simulink model "DDCU_wxt_v02_forA_OpenLoop"  (R2014a)
settings: Solver=FixedStepDiscrete  StartTime=0.0  StopTime=16  FixedStep=0.05  RelTol=1e-3
InitFcn:
  | Veh_Par_wxt
values from neighbouring files (symbols this model uses):
  ag_thr = 0.4*g    (= 3.924)    [Veh_Par_wxt.m]
  B = 2.25    [Veh_Par_wxt.m]
  bra_pre_em = 12    [Veh_Par_wxt.m]
  bra_pre_gz2 = 12/3    (= 4)    [Veh_Par_wxt.m]
  bra_pre_gz34 = 12/3    (= 4)    [Veh_Par_wxt.m]
  bra_pre_yd = 12/2    (= 6)    [Veh_Par_wxt.m]
  brakepre_dem_data = [0 1 2 3 4 5 6 7 8 9 10 11 12]    [Veh_Par_wxt.m]
  brakeTrq_dem_data = [0 218.198 436.396 654.594 872.792 1090.99 1309.188 1527.386 1745.584 1963.782 2181.98 2400.178 2618.376]    [Veh_Par_wxt.m]
  bratrq_max = 4*2618.376    (= 10473.504)    [Veh_Par_wxt.m]
  eff_tran = 0.75    [Veh_Par_wxt.m]
  G = Mass*g    (= 36297)    [Veh_Par_wxt.m]
  kd1 = 1    [Veh_Par_wxt.m]
  kd2 = 1    [Veh_Par_wxt.m]
  kd3 = 1    [Veh_Par_wxt.m]
  ki1 = 1    [Veh_Par_wxt.m]
  ki2 = 1    [Veh_Par_wxt.m]
  ki3 = 1    [Veh_Par_wxt.m]
  kp1 = 1    [Veh_Par_wxt.m]
  kp2 = 1    [Veh_Par_wxt.m]
  kp3 = 1    [Veh_Par_wxt.m]
  L = 3.12    [Veh_Par_wxt.m]
  premax = 12    [Veh_Par_wxt.m]
  Radius = 0.20    (= 0.2)    [Veh_Par_wxt.m]
  s_opt_yi_add = 0.05    [Veh_Par_wxt.m]
  s_opt_zhuan_add = 0.05    [Veh_Par_wxt.m]
  spd_map_mot = [0 100 200 300 360 400 500 600 700 800 900]*tras_ratio    [Veh_Par_wxt.m]
  spdmax = 900*tras_ratio    (= 5580)    [Veh_Par_wxt.m]
  speed_thr_park = 5/3.6/Radius*30/pi    (= 66.3145596216)    [Veh_Par_wxt.m]
  tras_ratio = 6.2    [Veh_Par_wxt.m]
  trq_map_mot = [1200 1200 1200 1200 1200 1080 864 720 617 540 480]/tras_ratio    [Veh_Par_wxt.m]
  trqmax = 80    [Veh_Par_wxt.m]
  v_thr1_b = 5    [Veh_Par_wxt.m]
  v_thr2_b = 20    [Veh_Par_wxt.m]
  v_thr_park = 5    [Veh_Par_wxt.m]
undefined symbols (not defined in the file or in its folder): DiscIntNeverNeededParam, sigbuilder_block
libraries: simulink x169, ec5744lib x9
(part 3 of 13)

== system DDCU_wxt_v02_forA_OpenLoop/OutputSignalProcess/VCU_ESC/VVMS_BrkPSetLe_MPa ==
  VVMS_BrkPSetLe_MPa : Inport
  Constant{2..8} (7 alike) : Constant  Value=0  OutDataTypeStr=uint8
  VVMS_BrkPSetLe_MPaRon : Rounding  Operator=round
  VVMS_BrkPSetLe_MPa_1sat : Saturate  UpperLimit=255  LowerLimit=0
  VVMS_BrkPSetLe_MPa_Convert : DataTypeConversion  OutDataTypeStr=uint8
  VVMS_BrkPSetLe_MPa_Convert1 : DataTypeConversion  OutDataTypeStr=uint32
  VVMS_BrkPSetLe_MPa_D : Product  Inputs=*/
  VVMS_BrkPSetLe_MPa_F : Constant  Value=0.1  OutDataTypeStr=single
  VVMS_BrkPSetLe_MPa_L : simulink/Logic and Bit Operations/Bitwise Operator  logicop=AND  UseBitMask=on  BitMask=255  BitMaskRealWorld=Stored Integer
  VVMS_BrkPSetLe_MPa_O : Constant  Value=0  OutDataTypeStr=single
  VVMS_BrkPSetLe_MPa_S : ArithShift
  VVMS_BrkPSetLe_MPa_sat : Saturate  UpperLimit=25.5  LowerLimit=0
  VVMS_BrkPSetLe_MPa_st : Sum  Inputs=+-
  output1 : Outport
  output2 : Outport  Port=2
  output3 : Outport  Port=3
  output4 : Outport  Port=4
  output5 : Outport  Port=5
  output6 : Outport  Port=6
  output7 : Outport  Port=7
  output8 : Outport  Port=8
  wires:
  VVMS_BrkPSetLe_MPa/1 -> VVMS_BrkPSetLe_MPa_sat/1
  VVMS_BrkPSetLe_MPa_sat/1 -> VVMS_BrkPSetLe_MPa_st/1
  VVMS_BrkPSetLe_MPa_O/1 -> VVMS_BrkPSetLe_MPa_st/2
  VVMS_BrkPSetLe_MPa_st/1 -> VVMS_BrkPSetLe_MPa_D/1
  VVMS_BrkPSetLe_MPa_F/1 -> VVMS_BrkPSetLe_MPa_D/2
  VVMS_BrkPSetLe_MPa_D/1 -> VVMS_BrkPSetLe_MPaRon/1
  VVMS_BrkPSetLe_MPaRon/1 -> VVMS_BrkPSetLe_MPa_S/1
  VVMS_BrkPSetLe_MPa_S/1 -> VVMS_BrkPSetLe_MPa_1sat/1
  VVMS_BrkPSetLe_MPa_1sat/1 -> VVMS_BrkPSetLe_MPa_Convert1/1
  VVMS_BrkPSetLe_MPa_Convert1/1 -> VVMS_BrkPSetLe_MPa_L/1
  VVMS_BrkPSetLe_MPa_L/1 -> VVMS_BrkPSetLe_MPa_Convert/1
  VVMS_BrkPSetLe_MPa_Convert/1 -> output1/1
  Constant2/1 -> output2/1
  Constant3/1 -> output3/1
  Constant4/1 -> output4/1
  Constant5/1 -> output5/1
  Constant6/1 -> output6/1
  Constant7/1 -> output7/1
  Constant8/1 -> output8/1

== system DDCU_wxt_v02_forA_OpenLoop/OutputSignalProcess/VCU_ESC/VVMS_BrkPSetRi_MPa ==
  VVMS_BrkPSetRi_MPa : Inport
  Constant{1,3..8} (7 alike) : Constant  Value=0  OutDataTypeStr=uint8
  VVMS_BrkPSetRi_MPaRon : Rounding  Operator=round
  VVMS_BrkPSetRi_MPa_1sat : Saturate  UpperLimit=255  LowerLimit=0
  VVMS_BrkPSetRi_MPa_Convert : DataTypeConversion  OutDataTypeStr=uint8
  VVMS_BrkPSetRi_MPa_Convert1 : DataTypeConversion  OutDataTypeStr=uint32
  VVMS_BrkPSetRi_MPa_D : Product  Inputs=*/
  VVMS_BrkPSetRi_MPa_F : Constant  Value=0.1  OutDataTypeStr=single
  VVMS_BrkPSetRi_MPa_L : simulink/Logic and Bit Operations/Bitwise Operator  logicop=AND  UseBitMask=on  BitMask=255  BitMaskRealWorld=Stored Integer
  VVMS_BrkPSetRi_MPa_O : Constant  Value=0  OutDataTypeStr=single
  VVMS_BrkPSetRi_MPa_S : ArithShift
  VVMS_BrkPSetRi_MPa_sat : Saturate  UpperLimit=25.5  LowerLimit=0
  VVMS_BrkPSetRi_MPa_st : Sum  Inputs=+-
  output1 : Outport
  output2 : Outport  Port=2
  output3 : Outport  Port=3
  output4 : Outport  Port=4
  output5 : Outport  Port=5
  output6 : Outport  Port=6
  output7 : Outport  Port=7
  output8 : Outport  Port=8
  wires:
  VVMS_BrkPSetRi_MPa/1 -> VVMS_BrkPSetRi_MPa_sat/1
  VVMS_BrkPSetRi_MPa_sat/1 -> VVMS_BrkPSetRi_MPa_st/1
  VVMS_BrkPSetRi_MPa_O/1 -> VVMS_BrkPSetRi_MPa_st/2
  VVMS_BrkPSetRi_MPa_st/1 -> VVMS_BrkPSetRi_MPa_D/1
  VVMS_BrkPSetRi_MPa_F/1 -> VVMS_BrkPSetRi_MPa_D/2
  VVMS_BrkPSetRi_MPa_D/1 -> VVMS_BrkPSetRi_MPaRon/1
  VVMS_BrkPSetRi_MPaRon/1 -> VVMS_BrkPSetRi_MPa_S/1
  VVMS_BrkPSetRi_MPa_S/1 -> VVMS_BrkPSetRi_MPa_1sat/1
  VVMS_BrkPSetRi_MPa_1sat/1 -> VVMS_BrkPSetRi_MPa_Convert1/1
  VVMS_BrkPSetRi_MPa_Convert1/1 -> VVMS_BrkPSetRi_MPa_L/1
  VVMS_BrkPSetRi_MPa_L/1 -> VVMS_BrkPSetRi_MPa_Convert/1
  VVMS_BrkPSetRi_MPa_Convert/1 -> output2/1
  Constant1/1 -> output1/1
  Constant3/1 -> output3/1
  Constant4/1 -> output4/1
  Constant5/1 -> output5/1
  Constant6/1 -> output6/1
  Constant7/1 -> output7/1
  Constant8/1 -> output8/1

== system DDCU_wxt_v02_forA_OpenLoop/OutputSignalProcess/VCU_ESC/VVMS_BrkSts_flg ==
  VVMS_BrkSts_flg : Inport
  Constant{1..2,4..8} (7 alike) : Constant  Value=0  OutDataTypeStr=uint8
  VVMS_BrkSts_flgRon : Rounding  Operator=round
  VVMS_BrkSts_flg_1sat : Saturate  UpperLimit=64  LowerLimit=0
  VVMS_BrkSts_flg_Convert : DataTypeConversion  OutDataTypeStr=uint8
  VVMS_BrkSts_flg_Convert1 : DataTypeConversion  OutDataTypeStr=uint32
  VVMS_BrkSts_flg_D : Product  Inputs=*/
  VVMS_BrkSts_flg_F : Constant  OutDataTypeStr=single
  VVMS_BrkSts_flg_L : simulink/Logic and Bit Operations/Bitwise Operator  logicop=AND  UseBitMask=on  BitMask=64  BitMaskRealWorld=Stored Integer
  VVMS_BrkSts_flg_O : Constant  Value=0  OutDataTypeStr=single
  VVMS_BrkSts_flg_S : ArithShift  BitShiftNumber=-6
  VVMS_BrkSts_flg_sat : Saturate  UpperLimit=1  LowerLimit=0
  VVMS_BrkSts_flg_st : Sum  Inputs=+-
  output1 : Outport
  output2 : Outport  Port=2
  output3 : Outport  Port=3
  output4 : Outport  Port=4
  output5 : Outport  Port=5
  output6 : Outport  Port=6
  output7 : Outport  Port=7
  output8 : Outport  Port=8
  wires:
  VVMS_BrkSts_flg/1 -> VVMS_BrkSts_flg_sat/1
  VVMS_BrkSts_flg_sat/1 -> VVMS_BrkSts_flg_st/1
  VVMS_BrkSts_flg_O/1 -> VVMS_BrkSts_flg_st/2
  VVMS_BrkSts_flg_st/1 -> VVMS_BrkSts_flg_D/1
  VVMS_BrkSts_flg_F/1 -> VVMS_BrkSts_flg_D/2
  VVMS_BrkSts_flg_D/1 -> VVMS_BrkSts_flgRon/1
  VVMS_BrkSts_flgRon/1 -> VVMS_BrkSts_flg_S/1
  VVMS_BrkSts_flg_S/1 -> VVMS_BrkSts_flg_1sat/1
  VVMS_BrkSts_flg_1sat/1 -> VVMS_BrkSts_flg_Convert1/1
  VVMS_BrkSts_flg_Convert1/1 -> VVMS_BrkSts_flg_L/1
  VVMS_BrkSts_flg_L/1 -> VVMS_BrkSts_flg_Convert/1
  VVMS_BrkSts_flg_Convert/1 -> output3/1
  Constant1/1 -> output1/1
  Constant2/1 -> output2/1
  Constant4/1 -> output4/1
  Constant5/1 -> output5/1
  Constant6/1 -> output6/1
  Constant7/1 -> output7/1
  Constant8/1 -> output8/1

== system DDCU_wxt_v02_forA_OpenLoop/OutputSignalProcess/VCU_ESC/VVMS_ParkSts_flg ==
  VVMS_ParkSts_flg : Inport
  Constant{1..2,4..8} (7 alike) : Constant  Value=0  OutDataTypeStr=uint8
  VVMS_ParkSts_flgRon : Rounding  Operator=round
  VVMS_ParkSts_flg_1sat : Saturate  UpperLimit=128  LowerLimit=0
  VVMS_ParkSts_flg_Convert : DataTypeConversion  OutDataTypeStr=uint8
  VVMS_ParkSts_flg_Convert1 : DataTypeConversion  OutDataTypeStr=uint32
  VVMS_ParkSts_flg_D : Product  Inputs=*/
  VVMS_ParkSts_flg_F : Constant  OutDataTypeStr=single
  VVMS_ParkSts_flg_L : simulink/Logic and Bit Operations/Bitwise Operator  logicop=AND  UseBitMask=on  BitMask=128  BitMaskRealWorld=Stored Integer
  VVMS_ParkSts_flg_O : Constant  Value=0  OutDataTypeStr=single
  VVMS_ParkSts_flg_S : ArithShift  BitShiftNumber=-7
  VVMS_ParkSts_flg_sat : Saturate  UpperLimit=1  LowerLimit=0
  VVMS_ParkSts_flg_st : Sum  Inputs=+-
  output1 : Outport
  output2 : Outport  Port=2
  output3 : Outport  Port=3
  output4 : Outport  Port=4
  output5 : Outport  Port=5
  output6 : Outport  Port=6
  output7 : Outport  Port=7
  output8 : Outport  Port=8
  wires:
  VVMS_ParkSts_flg/1 -> VVMS_ParkSts_flg_sat/1
  VVMS_ParkSts_flg_sat/1 -> VVMS_ParkSts_flg_st/1
  VVMS_ParkSts_flg_O/1 -> VVMS_ParkSts_flg_st/2
  VVMS_ParkSts_flg_st/1 -> VVMS_ParkSts_flg_D/1
  VVMS_ParkSts_flg_F/1 -> VVMS_ParkSts_flg_D/2
  VVMS_ParkSts_flg_D/1 -> VVMS_ParkSts_flgRon/1
  VVMS_ParkSts_flgRon/1 -> VVMS_ParkSts_flg_S/1
  VVMS_ParkSts_flg_S/1 -> VVMS_ParkSts_flg_1sat/1
  VVMS_ParkSts_flg_1sat/1 -> VVMS_ParkSts_flg_Convert1/1
  VVMS_ParkSts_flg_Convert1/1 -> VVMS_ParkSts_flg_L/1
  VVMS_ParkSts_flg_L/1 -> VVMS_ParkSts_flg_Convert/1
  VVMS_ParkSts_flg_Convert/1 -> output3/1
  Constant1/1 -> output1/1
  Constant2/1 -> output2/1
  Constant4/1 -> output4/1
  Constant5/1 -> output5/1
  Constant6/1 -> output6/1
  Constant7/1 -> output7/1
  Constant8/1 -> output8/1

== system DDCU_wxt_v02_forA_OpenLoop/OutputSignalProcess/VCU_MCU1/M1Drive ==
  M1Drive : Inport
  Constant{2..8} (7 alike) : Constant  Value=0  OutDataTypeStr=uint8
  M1DriveRon : Rounding  Operator=round
  M1Drive_1sat : Saturate  UpperLimit=48  LowerLimit=0
  M1Drive_Convert : DataTypeConversion  OutDataTypeStr=uint8
  M1Drive_Convert1 : DataTypeConversion  OutDataTypeStr=uint32
  M1Drive_D : Product  Inputs=*/
  M1Drive_F : Constant  OutDataTypeStr=single
  M1Drive_L : simulink/Logic and Bit Operations/Bitwise Operator  logicop=AND  UseBitMask=on  BitMask=48  BitMaskRealWorld=Stored Integer
  M1Drive_O : Constant  Value=0  OutDataTypeStr=single
  M1Drive_S : ArithShift  BitShiftNumber=-4
  M1Drive_sat : Saturate  UpperLimit=3  LowerLimit=0
  M1Drive_st : Sum  Inputs=+-
  output1 : Outport
  output2 : Outport  Port=2
  output3 : Outport  Port=3
  output4 : Outport  Port=4
  output5 : Outport  Port=5
  output6 : Outport  Port=6
  output7 : Outport  Port=7
  output8 : Outport  Port=8
  wires:
  M1Drive/1 -> M1Drive_sat/1
  M1Drive_sat/1 -> M1Drive_st/1
  M1Drive_O/1 -> M1Drive_st/2
  M1Drive_st/1 -> M1Drive_D/1
  M1Drive_F/1 -> M1Drive_D/2
  M1Drive_D/1 -> M1DriveRon/1
  M1DriveRon/1 -> M1Drive_S/1
  M1Drive_S/1 -> M1Drive_1sat/1
  M1Drive_1sat/1 -> M1Drive_Convert1/1
  M1Drive_Convert1/1 -> M1Drive_L/1
  M1Drive_L/1 -> M1Drive_Convert/1
  M1Drive_Convert/1 -> output1/1
  Constant2/1 -> output2/1
  Constant3/1 -> output3/1
  Constant4/1 -> output4/1
  Constant5/1 -> output5/1
  Constant6/1 -> output6/1
  Constant7/1 -> output7/1
  Constant8/1 -> output8/1

== system DDCU_wxt_v02_forA_OpenLoop/OutputSignalProcess/VCU_MCU1/M1Enable ==
  M1Enable : Inport
  Constant{2..8} (7 alike) : Constant  Value=0  OutDataTypeStr=uint8
  M1EnableRon : Rounding  Operator=round
  M1Enable_1sat : Saturate  UpperLimit=3  LowerLimit=0
  M1Enable_Convert : DataTypeConversion  OutDataTypeStr=uint8
  M1Enable_Convert1 : DataTypeConversion  OutDataTypeStr=uint32
  M1Enable_D : Product  Inputs=*/
  M1Enable_F : Constant  OutDataTypeStr=single
  M1Enable_L : simulink/Logic and Bit Operations/Bitwise Operator  logicop=AND  UseBitMask=on  BitMask=3  BitMaskRealWorld=Stored Integer
  M1Enable_O : Constant  Value=0  OutDataTypeStr=single
  M1Enable_S : ArithShift
  M1Enable_sat : Saturate  UpperLimit=3  LowerLimit=0
  M1Enable_st : Sum  Inputs=+-
  output1 : Outport
  output2 : Outport  Port=2
  output3 : Outport  Port=3
  output4 : Outport  Port=4
  output5 : Outport  Port=5
  output6 : Outport  Port=6
  output7 : Outport  Port=7
  output8 : Outport  Port=8
  wires:
  M1Enable/1 -> M1Enable_sat/1
  M1Enable_sat/1 -> M1Enable_st/1
  M1Enable_O/1 -> M1Enable_st/2
  M1Enable_st/1 -> M1Enable_D/1
  M1Enable_F/1 -> M1Enable_D/2
  M1Enable_D/1 -> M1EnableRon/1
  M1EnableRon/1 -> M1Enable_S/1
  M1Enable_S/1 -> M1Enable_1sat/1
  M1Enable_1sat/1 -> M1Enable_Convert1/1
  M1Enable_Convert1/1 -> M1Enable_L/1
  M1Enable_L/1 -> M1Enable_Convert/1
  M1Enable_Convert/1 -> output1/1
  Constant2/1 -> output2/1
  Constant3/1 -> output3/1
  Constant4/1 -> output4/1
  Constant5/1 -> output5/1
  Constant6/1 -> output6/1
  Constant7/1 -> output7/1
  Constant8/1 -> output8/1

== system DDCU_wxt_v02_forA_OpenLoop/OutputSignalProcess/VCU_MCU1/M1Mode ==
  M1Mode : Inport
  Constant{2..8} (7 alike) : Constant  Value=0  OutDataTypeStr=uint8
  M1ModeRon : Rounding  Operator=round
  M1Mode_1sat : Saturate  UpperLimit=12  LowerLimit=0
  M1Mode_Convert : DataTypeConversion  OutDataTypeStr=uint8
  M1Mode_Convert1 : DataTypeConversion  OutDataTypeStr=uint32
  M1Mode_D : Product  Inputs=*/
  M1Mode_F : Constant  OutDataTypeStr=single
  M1Mode_L : simulink/Logic and Bit Operations/Bitwise Operator  logicop=AND  UseBitMask=on  BitMask=12  BitMaskRealWorld=Stored Integer
  M1Mode_O : Constant  Value=0  OutDataTypeStr=single
  M1Mode_S : ArithShift  BitShiftNumber=-2
  M1Mode_sat : Saturate  UpperLimit=3  LowerLimit=0
  M1Mode_st : Sum  Inputs=+-
  output1 : Outport
  output2 : Outport  Port=2
  output3 : Outport  Port=3
  output4 : Outport  Port=4
  output5 : Outport  Port=5
  output6 : Outport  Port=6
  output7 : Outport  Port=7
  output8 : Outport  Port=8
  wires:
  M1Mode/1 -> M1Mode_sat/1
  M1Mode_sat/1 -> M1Mode_st/1
  M1Mode_O/1 -> M1Mode_st/2
  M1Mode_st/1 -> M1Mode_D/1
  M1Mode_F/1 -> M1Mode_D/2
  M1Mode_D/1 -> M1ModeRon/1
  M1ModeRon/1 -> M1Mode_S/1
  M1Mode_S/1 -> M1Mode_1sat/1
  M1Mode_1sat/1 -> M1Mode_Convert1/1
  M1Mode_Convert1/1 -> M1Mode_L/1
  M1Mode_L/1 -> M1Mode_Convert/1
  M1Mode_Convert/1 -> output1/1
  Constant2/1 -> output2/1
  Constant3/1 -> output3/1
  Constant4/1 -> output4/1
  Constant5/1 -> output5/1
  Constant6/1 -> output6/1
  Constant7/1 -> output7/1
  Constant8/1 -> output8/1

== system DDCU_wxt_v02_forA_OpenLoop/OutputSignalProcess/VCU_MCU1/M1SpeedLimit ==
  M1SpeedLimit : Inport
  BitCov : DataTypeConversion  OutDataTypeStr=uint8
  Constant{1..2,5..8} (6 alike) : Constant  Value=0  OutDataTypeStr=uint8
  M1SpeedLimitCOV : DataTypeConversion  OutDataTypeStr=uint8
  M1SpeedLimitRon : Rounding  Operator=round
  M1SpeedLimit_1sat : Saturate  UpperLimit=16380  LowerLimit=0
  M1SpeedLimit_And : simulink/Logic and Bit Operations/Bitwise Operator  logicop=AND  UseBitMask=off  NumInputPorts=2  BitMask=bin2dec('11011001')  BitMaskRealWorld=Stored Integer
  M1SpeedLimit_And_C : Constant  Value=255  OutDataTypeStr=uint32
  M1SpeedLimit_Convert : DataTypeConversion  OutDataTypeStr=uint32
  M1SpeedLimit_D : Product  Inputs=*/
  M1SpeedLimit_D1 : Product  Inputs=*/
  M1SpeedLimit_F : Constant  Value=5  OutDataTypeStr=single
  M1SpeedLimit_L : simulink/Logic and Bit Operations/Bitwise Operator  logicop=AND  UseBitMask=on  BitMask=16380  BitMaskRealWorld=Stored Integer
  M1SpeedLimit_O : Constant  Value=0  OutDataTypeStr=single
  M1SpeedLimit_S : ArithShift  BitShiftNumber=-2
  M1SpeedLimit_sat : Saturate  UpperLimit=20475  LowerLimit=0
  M1SpeedLimit_st : Sum  Inputs=+-
  M1SpeedLimitoutput4_C : Constant  Value=256
  output1 : Outport
  output2 : Outport  Port=2
  output3 : Outport  Port=3
  output4 : Outport  Port=4
  output5 : Outport  Port=5
  output6 : Outport  Port=6
  output7 : Outport  Port=7
  output8 : Outport  Port=8
  wires:
  M1SpeedLimit/1 -> M1SpeedLimit_sat/1
  M1SpeedLimit_sat/1 -> M1SpeedLimit_st/1
  M1SpeedLimit_O/1 -> M1SpeedLimit_st/2
  M1SpeedLimit_st/1 -> M1SpeedLimit_D/1
  M1SpeedLimit_F/1 -> M1SpeedLimit_D/2
  M1SpeedLimit_D/1 -> M1SpeedLimitRon/1
  M1SpeedLimitRon/1 -> M1SpeedLimit_S/1
  M1SpeedLimit_S/1 -> M1SpeedLimit_1sat/1
  M1SpeedLimit_1sat/1 -> M1SpeedLimit_Convert/1
  M1SpeedLimit_Convert/1 -> M1SpeedLimit_L/1
  M1SpeedLimit_L/1 -> M1SpeedLimit_D1/1, M1SpeedLimit_And/1
  M1SpeedLimitoutput4_C/1 -> M1SpeedLimit_D1/2
  M1SpeedLimit_D1/1 -> M1SpeedLimitCOV/1
  M1SpeedLimitCOV/1 -> output4/1
  M1SpeedLimit_And_C/1 -> M1SpeedLimit_And/2
  M1SpeedLimit_And/1 -> BitCov/1
  BitCov/1 -> output3/1
  Constant1/1 -> output1/1
  Constant2/1 -> output2/1
  Constant5/1 -> output5/1
  Constant6/1 -> output6/1
  Constant7/1 -> output7/1
  Constant8/1 -> output8/1

== matlab function DDCU_wxt_v02_forA_OpenLoop/MainControl/mode_control/forward/forward/Drive/驱动防滑控制TCS/直行TCS/直行/MATLAB Function3 ==
  data: s_act_rr input; flag_rr output; s_opt_zhuan input; s_opt_zhuan_add input; flag_rr_pre input
function flag_rr = fcn(s_act_rr,s_opt_zhuan,s_opt_zhuan_add,flag_rr_pre)
%#codegen
if s_act_rr>s_opt_zhuan+s_opt_zhuan_add
    flag_rr=1;
elseif s_act_rr<s_opt_zhuan
    flag_rr = 0;
else
    flag_rr=flag_rr_pre;
end
end

== matlab function DDCU_wxt_v02_forA_OpenLoop/MainControl/mode_control/forward/forward/Drive/驱动防滑控制TCS/直行TCS/直行/HeartBeat ==
  data: life_pre input; life output
function life = fcn(life_pre)
%#codegen
life=life_pre+1;
if life>15
    life=0;
end
end

== matlab function DDCU_wxt_v02_forA_OpenLoop/MainControl/mode_control/backward/backward/Brake/MATLAB Function3 ==
  data: syi_act_rf input; flagyi_rf output; s_opt_yi input; s_opt_yi_add input; flagyi_rf_pre input
function flagyi_rf = fcn(syi_act_rf,s_opt_yi,s_opt_yi_add,flagyi_rf_pre)
%#codegen
if syi_act_rf>s_opt_yi+s_opt_yi_add
    flagyi_rf=1;
elseif syi_act_rf<s_opt_yi
    flagyi_rf = 0;
else
    flagyi_rf=flagyi_rf_pre;
end
end

== matlab function DDCU_wxt_v02_forA_OpenLoop/MainControl/mode_control/backward/backward/Drive/目标转向力矩确定模块/MATLAB Function1 ==
  data: v_act input; Rturn_min_ag output; ag_thr input
function Rturn_min_ag = fcn(v_act,ag_thr)
%#codegen

    Rturn_min_ag=(v_act/3.6)^2/ag_thr;
end

== matlab function DDCU_wxt_v02_forA_OpenLoop/MainControl/mode_control/backward/backward/Drive/驱动防滑控制TCS/直行TCS/直行/HeartBeat ==
  data: life_pre input; life output
function life = fcn(life_pre)
%#codegen
life=life_pre+1;
if life>15
    life=0;
end
end

== matlab function DDCU_wxt_v02_forA_OpenLoop/MainControl/mode_control/backward/backward/Drive/驱动防滑控制TCS/直行TCS/直行/MATLAB Function2 ==
  data: s_act_rf input; flag_rf output; s_opt_zhuan input; s_opt_zhuan_add input; flag_rf_pre input
function flag_rf = fcn(s_act_rf,s_opt_zhuan,s_opt_zhuan_add,flag_rf_pre)
%#codegen
if s_act_rf>s_opt_zhuan+s_opt_zhuan_add
    flag_rf=1;
elseif s_act_rf<s_opt_zhuan
    flag_rf = 0;
else
    flag_rf=flag_rf_pre;
end
end

== matlab function DDCU_wxt_v02_forA_OpenLoop/MainControl/mode_control/backward/backward/Drive/驱动防滑控制TCS/转向TCS/右转/MATLAB Function1 ==
  data: s_act_lr input; flag_lr output; s_opt_zhuan input; s_opt_zhuan_add input; flag_lr_pre input
function flag_lr = fcn(s_act_lr,s_opt_zhuan,s_opt_zhuan_add,flag_lr_pre)
%#codegen
if s_act_lr>s_opt_zhuan+s_opt_zhuan_add
    flag_lr=1;
elseif s_act_lr<s_opt_zhuan
    flag_lr = 0;
else
    flag_lr=flag_lr_pre;
end
end

== matlab function DDCU_wxt_v02_forA_OpenLoop/MainControl/mode_control/backward/backward/Drive/驱动防滑控制TCS/转向TCS/右转/前后轮均滑转/HeartBeat ==
  data: life_pre input; life output
function life = fcn(life_pre)
%#codegen
life=life_pre+1;
if life>15
    life=0;
end
end

== matlab function DDCU_wxt_v02_forA_OpenLoop/MainControl/mode_control/backward/backward/Drive/驱动防滑控制TCS/转向TCS/右转/前轮滑转/HeartBeat1 ==
  data: life_pre input; life output
function life = fcn(life_pre)
%#codegen
life=life_pre+1;
if life>15
    life=0;
end
end

== matlab function DDCU_wxt_v02_forA_OpenLoop/MainControl/mode_control/backward/backward/Drive/驱动防滑控制TCS/转向TCS/右转/无滑转/HeartBeat1 ==
  data: life_pre input; life output
function life = fcn(life_pre)
%#codegen
life=life_pre+1;
if life>15
    life=0;
end
end

== matlab function DDCU_wxt_v02_forA_OpenLoop/MainControl/mode_control/backward/backward/Drive/驱动防滑控制TCS/转向TCS/左转/MATLAB Function3 ==
  data: s_act_rr input; flag_rr output; s_opt_zhuan input; s_opt_zhuan_add input; flag_rr_pre input
function flag_rr = fcn(s_act_rr,s_opt_zhuan,s_opt_zhuan_add,flag_rr_pre)
%#codegen
if s_act_rr>s_opt_zhuan+s_opt_zhuan_add
    flag_rr=1;
elseif s_act_rr<s_opt_zhuan
    flag_rr = 0;
else
    flag_rr=flag_rr_pre;
end
end

== matlab function DDCU_wxt_v02_forA_OpenLoop/MainControl/mode_control/backward/backward/Drive/驱动防滑控制TCS/转向TCS/左转/前轮滑转/HeartBeat ==
  data: life_pre input; life output
function life = fcn(life_pre)
%#codegen
life=life_pre+1;
if life>15
    life=0;
end
end

== matlab function DDCU_wxt_v02_forA_OpenLoop/MainControl/mode_control/backward/backward/Drive/驱动防滑控制TCS/转向TCS/左转/无滑转/HeartBeat ==
  data: life_pre input; life output
function life = fcn(life_pre)
%#codegen
life=life_pre+1;
if life>15
    life=0;
end
end

== system DDCU_wxt_v02_forA_OpenLoop/OutputSignalProcess/VCU_MCU1/M1TorqueSet ==
  M1TorqueSet : Inport
  Constant{4..8} (5 alike) : Constant  Value=0  OutDataTypeStr=uint8
  M1TorqueSetBitCov : DataTypeConversion  OutDataTypeStr=uint32
  M1TorqueSetBitCov1 : DataTypeConversion  OutDataTypeStr=uint8
  M1TorqueSetCOV : DataTypeConversion  OutDataTypeStr=uint8
  M1TorqueSetCOV1 : DataTypeConversion  OutDataTypeStr=uint8
  M1TorqueSetRon : Rounding  Operator=round
  M1TorqueSet_1sat : Saturate  UpperLimit=262080  LowerLimit=0
  M1TorqueSet_And : simulink/Logic and Bit Operations/Bitwise Operator  logicop=AND  UseBitMask=off  NumInputPorts=2  BitMask=bin2dec('11011001')  BitMaskRealWorld=Stored Integer
  M1TorqueSet_And1 : simulink/Logic and Bit Operations/Bitwise Operator  logicop=AND  UseBitMask=off  NumInputPorts=2  BitMask=bin2dec('11011001')  BitMaskRealWorld=Stored Integer
  M1TorqueSet_And1_C : Constant  Value=255  OutDataTypeStr=uint32
  M1TorqueSet_And_C : Constant  Value=65535
  M1TorqueSet_Convert : DataTypeConversion  OutDataTypeStr=uint32
  M1TorqueSet_D : Product  Inputs=*/
  M1TorqueSet_D1 : Product  Inputs=*/
  M1TorqueSet_D2 : Product  Inputs=*/
  M1TorqueSet_F : Constant  Value=0.25  OutDataTypeStr=single
  M1TorqueSet_L : simulink/Logic and Bit Operations/Bitwise Operator  logicop=AND  UseBitMask=on  BitMask=262080  BitMaskRealWorld=Stored Integer
  M1TorqueSet_O : Constant  Value=-300  OutDataTypeStr=single
  M1TorqueSet_S : ArithShift  BitShiftNumber=-6
  M1TorqueSet_sat : Saturate  UpperLimit=723.75  LowerLimit=-300
  M1TorqueSet_st : Sum  Inputs=+-
  M1TorqueSetoutput2_C : Constant  Value=256
  M1TorqueSetoutput3_C : Constant  Value=65536
  output1 : Outport
  output2 : Outport  Port=2
  output3 : Outport  Port=3
  output4 : Outport  Port=4
  output5 : Outport  Port=5
  output6 : Outport  Port=6
  output7 : Outport  Port=7
  output8 : Outport  Port=8
  wires:
  M1TorqueSet/1 -> M1TorqueSet_sat/1
  M1TorqueSet_sat/1 -> M1TorqueSet_st/1
  M1TorqueSet_O/1 -> M1TorqueSet_st/2
  M1TorqueSet_st/1 -> M1TorqueSet_D/1
  M1TorqueSet_F/1 -> M1TorqueSet_D/2
  M1TorqueSet_D/1 -> M1TorqueSetRon/1
  M1TorqueSetRon/1 -> M1TorqueSet_S/1
  M1TorqueSet_S/1 -> M1TorqueSet_1sat/1
  M1TorqueSet_1sat/1 -> M1TorqueSet_Convert/1
  M1TorqueSet_Convert/1 -> M1TorqueSet_L/1
  M1TorqueSet_L/1 -> M1TorqueSet_D1/1, M1TorqueSet_And/1, M1TorqueSet_And1/1
  M1TorqueSetoutput3_C/1 -> M1TorqueSet_D1/2
  M1TorqueSet_D1/1 -> M1TorqueSetCOV/1
  M1TorqueSetCOV/1 -> output3/1
  M1TorqueSet_And_C/1 -> M1TorqueSetBitCov/1
  M1TorqueSetBitCov/1 -> M1TorqueSet_And/2
  M1TorqueSet_And/1 -> M1TorqueSet_D2/1
  M1TorqueSetoutput2_C/1 -> M1TorqueSet_D2/2
  M1TorqueSet_D2/1 -> M1TorqueSetCOV1/1
  M1TorqueSetCOV1/1 -> output2/1
  M1TorqueSet_And1_C/1 -> M1TorqueSet_And1/2
  M1TorqueSet_And1/1 -> M1TorqueSetBitCov1/1
  M1TorqueSetBitCov1/1 -> output1/1
  Constant4/1 -> output4/1
  Constant5/1 -> output5/1
  Constant6/1 -> output6/1
  Constant7/1 -> output7/1
  Constant8/1 -> output8/1

== system DDCU_wxt_v02_forA_OpenLoop/OutputSignalProcess/VCU_MCU1/M2Drive ==
  M2Drive : Inport
  Constant{1..4,6..8} (7 alike) : Constant  Value=0  OutDataTypeStr=uint8
  M2DriveRon : Rounding  Operator=round
  M2Drive_1sat : Saturate  UpperLimit=12  LowerLimit=0
  M2Drive_Convert : DataTypeConversion  OutDataTypeStr=uint8
  M2Drive_Convert1 : DataTypeConversion  OutDataTypeStr=uint32
  M2Drive_D : Product  Inputs=*/
  M2Drive_F : Constant  OutDataTypeStr=single
  M2Drive_L : simulink/Logic and Bit Operations/Bitwise Operator  logicop=AND  UseBitMask=on  BitMask=12  BitMaskRealWorld=Stored Integer
  M2Drive_O : Constant  Value=0  OutDataTypeStr=single
  M2Drive_S : ArithShift  BitShiftNumber=-2
  M2Drive_sat : Saturate  UpperLimit=3  LowerLimit=0
  M2Drive_st : Sum  Inputs=+-
  output1 : Outport
  output2 : Outport  Port=2
  output3 : Outport  Port=3
  output4 : Outport  Port=4
  output5 : Outport  Port=5
  output6 : Outport  Port=6
  output7 : Outport  Port=7
  output8 : Outport  Port=8
  wires:
  M2Drive/1 -> M2Drive_sat/1
  M2Drive_sat/1 -> M2Drive_st/1
  M2Drive_O/1 -> M2Drive_st/2
  M2Drive_st/1 -> M2Drive_D/1
  M2Drive_F/1 -> M2Drive_D/2
  M2Drive_D/1 -> M2DriveRon/1
  M2DriveRon/1 -> M2Drive_S/1
  M2Drive_S/1 -> M2Drive_1sat/1
  M2Drive_1sat/1 -> M2Drive_Convert1/1
  M2Drive_Convert1/1 -> M2Drive_L/1
  M2Drive_L/1 -> M2Drive_Convert/1
  M2Drive_Convert/1 -> output5/1
  Constant1/1 -> output1/1
  Constant2/1 -> output2/1
  Constant3/1 -> output3/1
  Constant4/1 -> output4/1
  Constant6/1 -> output6/1
  Constant7/1 -> output7/1
  Constant8/1 -> output8/1

== system DDCU_wxt_v02_forA_OpenLoop/OutputSignalProcess/VCU_MCU1/M2Enable ==
  M2Enable : Inport
  Constant{1..3,5..8} (7 alike) : Constant  Value=0  OutDataTypeStr=uint8
  M2EnableRon : Rounding  Operator=round
  M2Enable_1sat : Saturate  UpperLimit=192  LowerLimit=0
  M2Enable_Convert : DataTypeConversion  OutDataTypeStr=uint8
  M2Enable_Convert1 : DataTypeConversion  OutDataTypeStr=uint32
  M2Enable_D : Product  Inputs=*/
  M2Enable_F : Constant  OutDataTypeStr=single
  M2Enable_L : simulink/Logic and Bit Operations/Bitwise Operator  logicop=AND  UseBitMask=on  BitMask=192  BitMaskRealWorld=Stored Integer
  M2Enable_O : Constant  Value=0  OutDataTypeStr=single
  M2Enable_S : ArithShift  BitShiftNumber=-6
  M2Enable_sat : Saturate  UpperLimit=3  LowerLimit=0
  M2Enable_st : Sum  Inputs=+-
  output1 : Outport
  output2 : Outport  Port=2
  output3 : Outport  Port=3
  output4 : Outport  Port=4
  output5 : Outport  Port=5
  output6 : Outport  Port=6
  output7 : Outport  Port=7
  output8 : Outport  Port=8
  wires:
  M2Enable/1 -> M2Enable_sat/1
  M2Enable_sat/1 -> M2Enable_st/1
  M2Enable_O/1 -> M2Enable_st/2
  M2Enable_st/1 -> M2Enable_D/1
  M2Enable_F/1 -> M2Enable_D/2
  M2Enable_D/1 -> M2EnableRon/1
  M2EnableRon/1 -> M2Enable_S/1
  M2Enable_S/1 -> M2Enable_1sat/1
  M2Enable_1sat/1 -> M2Enable_Convert1/1
  M2Enable_Convert1/1 -> M2Enable_L/1
  M2Enable_L/1 -> M2Enable_Convert/1
  M2Enable_Convert/1 -> output4/1
  Constant1/1 -> output1/1
  Constant2/1 -> output2/1
  Constant3/1 -> output3/1
  Constant5/1 -> output5/1
  Constant6/1 -> output6/1
  Constant7/1 -> output7/1
  Constant8/1 -> output8/1

== system DDCU_wxt_v02_forA_OpenLoop/OutputSignalProcess/VCU_MCU1/M2Mode ==
  M2Mode : Inport
  Constant{1..4,6..8} (7 alike) : Constant  Value=0  OutDataTypeStr=uint8
  M2ModeRon : Rounding  Operator=round
  M2Mode_1sat : Saturate  UpperLimit=3  LowerLimit=0
  M2Mode_Convert : DataTypeConversion  OutDataTypeStr=uint8
  M2Mode_Convert1 : DataTypeConversion  OutDataTypeStr=uint32
  M2Mode_D : Product  Inputs=*/
  M2Mode_F : Constant  OutDataTypeStr=single
  M2Mode_L : simulink/Logic and Bit Operations/Bitwise Operator  logicop=AND  UseBitMask=on  BitMask=3  BitMaskRealWorld=Stored Integer
  M2Mode_O : Constant  Value=0  OutDataTypeStr=single
  M2Mode_S : ArithShift
  M2Mode_sat : Saturate  UpperLimit=3  LowerLimit=0
  M2Mode_st : Sum  Inputs=+-
  output1 : Outport
  output2 : Outport  Port=2
  output3 : Outport  Port=3
  output4 : Outport  Port=4
  output5 : Outport  Port=5
  output6 : Outport  Port=6
  output7 : Outport  Port=7
  output8 : Outport  Port=8
  wires:
  M2Mode/1 -> M2Mode_sat/1
  M2Mode_sat/1 -> M2Mode_st/1
  M2Mode_O/1 -> M2Mode_st/2
  M2Mode_st/1 -> M2Mode_D/1
  M2Mode_F/1 -> M2Mode_D/2
  M2Mode_D/1 -> M2ModeRon/1
  M2ModeRon/1 -> M2Mode_S/1
  M2Mode_S/1 -> M2Mode_1sat/1
  M2Mode_1sat/1 -> M2Mode_Convert1/1
  M2Mode_Convert1/1 -> M2Mode_L/1
  M2Mode_L/1 -> M2Mode_Convert/1
  M2Mode_Convert/1 -> output5/1
  Constant1/1 -> output1/1
  Constant2/1 -> output2/1
  Constant3/1 -> output3/1
  Constant4/1 -> output4/1
  Constant6/1 -> output6/1
  Constant7/1 -> output7/1
  Constant8/1 -> output8/1

== system DDCU_wxt_v02_forA_OpenLoop/OutputSignalProcess/VCU_MCU1/M2SpeedLimit ==
  M2SpeedLimit : Inport
  Constant{1..6} (6 alike) : Constant  Value=0  OutDataTypeStr=uint8
  M2SpeedLimitBitCov : DataTypeConversion  OutDataTypeStr=uint8
  M2SpeedLimitCOV : DataTypeConversion  OutDataTypeStr=uint8
  M2SpeedLimitRon : Rounding  Operator=round
  M2SpeedLimit_1sat : Saturate  UpperLimit=4095  LowerLimit=0
  M2SpeedLimit_And : simulink/Logic and Bit Operations/Bitwise Operator  logicop=AND  UseBitMask=off  NumInputPorts=2  BitMask=bin2dec('11011001')  BitMaskRealWorld=Stored Integer
  M2SpeedLimit_And_C : Constant  Value=255  OutDataTypeStr=uint32
  M2SpeedLimit_Convert : DataTypeConversion  OutDataTypeStr=uint32
  M2SpeedLimit_D : Product  Inputs=*/
  M2SpeedLimit_D1 : Product  Inputs=*/
  M2SpeedLimit_F : Constant  Value=5  OutDataTypeStr=single
  M2SpeedLimit_L : simulink/Logic and Bit Operations/Bitwise Operator  logicop=AND  UseBitMask=on  BitMask=4095  BitMaskRealWorld=Stored Integer
  M2SpeedLimit_O : Constant  Value=0  OutDataTypeStr=single
  M2SpeedLimit_S : ArithShift
  M2SpeedLimit_sat : Saturate  UpperLimit=20475  LowerLimit=0
  M2SpeedLimit_st : Sum  Inputs=+-
  M2SpeedLimitoutput8_C : Constant  Value=256
  output1 : Outport
  output2 : Outport  Port=2
  output3 : Outport  Port=3
  output4 : Outport  Port=4
  output5 : Outport  Port=5
  output6 : Outport  Port=6
  output7 : Outport  Port=7
  output8 : Outport  Port=8
  wires:
  M2SpeedLimit/1 -> M2SpeedLimit_sat/1
  M2SpeedLimit_sat/1 -> M2SpeedLimit_st/1
  M2SpeedLimit_O/1 -> M2SpeedLimit_st/2
  M2SpeedLimit_st/1 -> M2SpeedLimit_D/1
  M2SpeedLimit_F/1 -> M2SpeedLimit_D/2
  M2SpeedLimit_D/1 -> M2SpeedLimitRon/1
  M2SpeedLimitRon/1 -> M2SpeedLimit_S/1
  M2SpeedLimit_S/1 -> M2SpeedLimit_1sat/1
  M2SpeedLimit_1sat/1 -> M2SpeedLimit_Convert/1
  M2SpeedLimit_Convert/1 -> M2SpeedLimit_L/1
  M2SpeedLimit_L/1 -> M2SpeedLimit_D1/1, M2SpeedLimit_And/1
  M2SpeedLimitoutput8_C/1 -> M2SpeedLimit_D1/2
  M2SpeedLimit_D1/1 -> M2SpeedLimitCOV/1
  M2SpeedLimitCOV/1 -> output8/1
  M2SpeedLimit_And_C/1 -> M2SpeedLimit_And/2
  M2SpeedLimit_And/1 -> M2SpeedLimitBitCov/1
  M2SpeedLimitBitCov/1 -> output7/1
  Constant1/1 -> output1/1
  Constant2/1 -> output2/1
  Constant3/1 -> output3/1
  Constant4/1 -> output4/1
  Constant5/1 -> output5/1
  Constant6/1 -> output6/1

== system DDCU_wxt_v02_forA_OpenLoop/OutputSignalProcess/VCU_MCU1/M2TorqueSet ==
  M2TorqueSet : Inport
  Constant{1..4,7..8} (6 alike) : Constant  Value=0  OutDataTypeStr=uint8
  M2TorqueSetBitCov : DataTypeConversion  OutDataTypeStr=uint8
  M2TorqueSetCOV : DataTypeConversion  OutDataTypeStr=uint8
  M2TorqueSetRon : Rounding  Operator=round
  M2TorqueSet_1sat : Saturate  UpperLimit=65520  LowerLimit=0
  M2TorqueSet_And : simulink/Logic and Bit Operations/Bitwise Operator  logicop=AND  UseBitMask=off  NumInputPorts=2  BitMask=bin2dec('11011001')  BitMaskRealWorld=Stored Integer
  M2TorqueSet_And_C : Constant  Value=255  OutDataTypeStr=uint32
  M2TorqueSet_Convert : DataTypeConversion  OutDataTypeStr=uint32
  M2TorqueSet_D : Product  Inputs=*/
  M2TorqueSet_D1 : Product  Inputs=*/
  M2TorqueSet_F : Constant  Value=0.25  OutDataTypeStr=single
  M2TorqueSet_L : simulink/Logic and Bit Operations/Bitwise Operator  logicop=AND  UseBitMask=on  BitMask=65520  BitMaskRealWorld=Stored Integer
  M2TorqueSet_O : Constant  Value=-300  OutDataTypeStr=single
  M2TorqueSet_S : ArithShift  BitShiftNumber=-4
  M2TorqueSet_sat : Saturate  UpperLimit=723.75  LowerLimit=-300
  M2TorqueSet_st : Sum  Inputs=+-
  M2TorqueSetoutput6_C : Constant  Value=256
  output1 : Outport
  output2 : Outport  Port=2
  output3 : Outport  Port=3
  output4 : Outport  Port=4
  output5 : Outport  Port=5
  output6 : Outport  Port=6
  output7 : Outport  Port=7
  output8 : Outport  Port=8
  wires:
  M2TorqueSet/1 -> M2TorqueSet_sat/1
  M2TorqueSet_sat/1 -> M2TorqueSet_st/1
  M2TorqueSet_O/1 -> M2TorqueSet_st/2
  M2TorqueSet_st/1 -> M2TorqueSet_D/1
  M2TorqueSet_F/1 -> M2TorqueSet_D/2
  M2TorqueSet_D/1 -> M2TorqueSetRon/1
  M2TorqueSetRon/1 -> M2TorqueSet_S/1
  M2TorqueSet_S/1 -> M2TorqueSet_1sat/1
  M2TorqueSet_1sat/1 -> M2TorqueSet_Convert/1
  M2TorqueSet_Convert/1 -> M2TorqueSet_L/1
  M2TorqueSet_L/1 -> M2TorqueSet_D1/1, M2TorqueSet_And/1
  M2TorqueSetoutput6_C/1 -> M2TorqueSet_D1/2
  M2TorqueSet_D1/1 -> M2TorqueSetCOV/1
  M2TorqueSetCOV/1 -> output6/1
  M2TorqueSet_And_C/1 -> M2TorqueSet_And/2
  M2TorqueSet_And/1 -> M2TorqueSetBitCov/1
  M2TorqueSetBitCov/1 -> output5/1
  Constant1/1 -> output1/1
  Constant2/1 -> output2/1
  Constant3/1 -> output3/1
  Constant4/1 -> output4/1
  Constant7/1 -> output7/1
  Constant8/1 -> output8/1

== system DDCU_wxt_v02_forA_OpenLoop/OutputSignalProcess/VCU_MCU1/MCU1HeartBeat ==
  MCU1HeartBeat : Inport
  Constant{1..7} (7 alike) : Constant  Value=0  OutDataTypeStr=uint8
  MCU1HeartBeatRon : Rounding  Operator=round
  MCU1HeartBeat_1sat : Saturate  UpperLimit=240  LowerLimit=0
  MCU1HeartBeat_Convert : DataTypeConversion  OutDataTypeStr=uint8
  MCU1HeartBeat_Convert1 : DataTypeConversion  OutDataTypeStr=uint32
  MCU1HeartBeat_D : Product  Inputs=*/
  MCU1HeartBeat_F : Constant  OutDataTypeStr=single
  MCU1HeartBeat_L : simulink/Logic and Bit Operations/Bitwise Operator  logicop=AND  UseBitMask=on  BitMask=240  BitMaskRealWorld=Stored Integer
  MCU1HeartBeat_O : Constant  Value=0  OutDataTypeStr=single
  MCU1HeartBeat_S : ArithShift  BitShiftNumber=-4
  MCU1HeartBeat_sat : Saturate  UpperLimit=15  LowerLimit=0
  MCU1HeartBeat_st : Sum  Inputs=+-
  output1 : Outport
  output2 : Outport  Port=2
  output3 : Outport  Port=3
  output4 : Outport  Port=4
  output5 : Outport  Port=5
  output6 : Outport  Port=6
  output7 : Outport  Port=7
  output8 : Outport  Port=8
  wires:
  MCU1HeartBeat/1 -> MCU1HeartBeat_sat/1
  MCU1HeartBeat_sat/1 -> MCU1HeartBeat_st/1
  MCU1HeartBeat_O/1 -> MCU1HeartBeat_st/2
  MCU1HeartBeat_st/1 -> MCU1HeartBeat_D/1
  MCU1HeartBeat_F/1 -> MCU1HeartBeat_D/2
  MCU1HeartBeat_D/1 -> MCU1HeartBeatRon/1
  MCU1HeartBeatRon/1 -> MCU1HeartBeat_S/1
  MCU1HeartBeat_S/1 -> MCU1HeartBeat_1sat/1
  MCU1HeartBeat_1sat/1 -> MCU1HeartBeat_Convert1/1
  MCU1HeartBeat_Convert1/1 -> MCU1HeartBeat_L/1
  MCU1HeartBeat_L/1 -> MCU1HeartBeat_Convert/1
  MCU1HeartBeat_Convert/1 -> output8/1
  Constant1/1 -> output1/1
  Constant2/1 -> output2/1
  Constant3/1 -> output3/1
  Constant4/1 -> output4/1
  Constant5/1 -> output5/1
  Constant6/1 -> output6/1
  Constant7/1 -> output7/1

== system DDCU_wxt_v02_forA_OpenLoop/OutputSignalProcess/VCU_MCU1_replace/M1Drive ==
  M1Drive : Inport
  Constant{2..8} (7 alike) : Constant  Value=0  OutDataTypeStr=uint8
  M1DriveRon : Rounding  Operator=round
  M1Drive_1sat : Saturate  UpperLimit=48  LowerLimit=0
  M1Drive_Convert : DataTypeConversion  OutDataTypeStr=uint8
  M1Drive_Convert1 : DataTypeConversion  OutDataTypeStr=uint32
  M1Drive_D : Product  Inputs=*/
  M1Drive_F : Constant  OutDataTypeStr=single
  M1Drive_L : simulink/Logic and Bit Operations/Bitwise Operator  logicop=AND  UseBitMask=on  BitMask=48  BitMaskRealWorld=Stored Integer
  M1Drive_O : Constant  Value=0  OutDataTypeStr=single
  M1Drive_S : ArithShift  BitShiftNumber=-4
  M1Drive_sat : Saturate  UpperLimit=3  LowerLimit=0
  M1Drive_st : Sum  Inputs=+-
  output1 : Outport
  output2 : Outport  Port=2
  output3 : Outport  Port=3
  output4 : Outport  Port=4
  output5 : Outport  Port=5
  output6 : Outport  Port=6
  output7 : Outport  Port=7
  output8 : Outport  Port=8
  wires:
  M1Drive/1 -> M1Drive_sat/1
  M1Drive_sat/1 -> M1Drive_st/1
  M1Drive_O/1 -> M1Drive_st/2
  M1Drive_st/1 -> M1Drive_D/1
  M1Drive_F/1 -> M1Drive_D/2
  M1Drive_D/1 -> M1DriveRon/1
  M1DriveRon/1 -> M1Drive_S/1
  M1Drive_S/1 -> M1Drive_1sat/1
  M1Drive_1sat/1 -> M1Drive_Convert1/1
  M1Drive_Convert1/1 -> M1Drive_L/1
  M1Drive_L/1 -> M1Drive_Convert/1
  M1Drive_Convert/1 -> output1/1
  Constant2/1 -> output2/1
  Constant3/1 -> output3/1
  Constant4/1 -> output4/1
  Constant5/1 -> output5/1
  Constant6/1 -> output6/1
  Constant7/1 -> output7/1
  Constant8/1 -> output8/1

== system DDCU_wxt_v02_forA_OpenLoop/OutputSignalProcess/VCU_MCU1_replace/M1Enable ==
  M1Enable : Inport
  Constant{2..8} (7 alike) : Constant  Value=0  OutDataTypeStr=uint8
  M1EnableRon : Rounding  Operator=round
  M1Enable_1sat : Saturate  UpperLimit=3  LowerLimit=0
  M1Enable_Convert : DataTypeConversion  OutDataTypeStr=uint8
  M1Enable_Convert1 : DataTypeConversion  OutDataTypeStr=uint32
  M1Enable_D : Product  Inputs=*/
  M1Enable_F : Constant  OutDataTypeStr=single
  M1Enable_L : simulink/Logic and Bit Operations/Bitwise Operator  logicop=AND  UseBitMask=on  BitMask=3  BitMaskRealWorld=Stored Integer
  M1Enable_O : Constant  Value=0  OutDataTypeStr=single
  M1Enable_S : ArithShift
  M1Enable_sat : Saturate  UpperLimit=3  LowerLimit=0
  M1Enable_st : Sum  Inputs=+-
  output1 : Outport
  output2 : Outport  Port=2
  output3 : Outport  Port=3
  output4 : Outport  Port=4
  output5 : Outport  Port=5
  output6 : Outport  Port=6
  output7 : Outport  Port=7
  output8 : Outport  Port=8
  wires:
  M1Enable/1 -> M1Enable_sat/1
  M1Enable_sat/1 -> M1Enable_st/1
  M1Enable_O/1 -> M1Enable_st/2
  M1Enable_st/1 -> M1Enable_D/1
  M1Enable_F/1 -> M1Enable_D/2
  M1Enable_D/1 -> M1EnableRon/1
  M1EnableRon/1 -> M1Enable_S/1
  M1Enable_S/1 -> M1Enable_1sat/1
  M1Enable_1sat/1 -> M1Enable_Convert1/1
  M1Enable_Convert1/1 -> M1Enable_L/1
  M1Enable_L/1 -> M1Enable_Convert/1
  M1Enable_Convert/1 -> output1/1
  Constant2/1 -> output2/1
  Constant3/1 -> output3/1
  Constant4/1 -> output4/1
  Constant5/1 -> output5/1
  Constant6/1 -> output6/1
  Constant7/1 -> output7/1
  Constant8/1 -> output8/1

== system DDCU_wxt_v02_forA_OpenLoop/OutputSignalProcess/VCU_MCU1_replace/M1Mode ==
  M1Mode : Inport
  Constant{2..8} (7 alike) : Constant  Value=0  OutDataTypeStr=uint8
  M1ModeRon : Rounding  Operator=round
  M1Mode_1sat : Saturate  UpperLimit=12  LowerLimit=0
  M1Mode_Convert : DataTypeConversion  OutDataTypeStr=uint8
  M1Mode_Convert1 : DataTypeConversion  OutDataTypeStr=uint32
  M1Mode_D : Product  Inputs=*/
  M1Mode_F : Constant  OutDataTypeStr=single
  M1Mode_L : simulink/Logic and Bit Operations/Bitwise Operator  logicop=AND  UseBitMask=on  BitMask=12  BitMaskRealWorld=Stored Integer
  M1Mode_O : Constant  Value=0  OutDataTypeStr=single
  M1Mode_S : ArithShift  BitShiftNumber=-2
  M1Mode_sat : Saturate  UpperLimit=3  LowerLimit=0
  M1Mode_st : Sum  Inputs=+-
  output1 : Outport
  output2 : Outport  Port=2
  output3 : Outport  Port=3
  output4 : Outport  Port=4
  output5 : Outport  Port=5
  output6 : Outport  Port=6
  output7 : Outport  Port=7
  output8 : Outport  Port=8
  wires:
  M1Mode/1 -> M1Mode_sat/1
  M1Mode_sat/1 -> M1Mode_st/1
  M1Mode_O/1 -> M1Mode_st/2
  M1Mode_st/1 -> M1Mode_D/1
  M1Mode_F/1 -> M1Mode_D/2
  M1Mode_D/1 -> M1ModeRon/1
  M1ModeRon/1 -> M1Mode_S/1
  M1Mode_S/1 -> M1Mode_1sat/1
  M1Mode_1sat/1 -> M1Mode_Convert1/1
  M1Mode_Convert1/1 -> M1Mode_L/1
  M1Mode_L/1 -> M1Mode_Convert/1
  M1Mode_Convert/1 -> output1/1
  Constant2/1 -> output2/1
  Constant3/1 -> output3/1
  Constant4/1 -> output4/1
  Constant5/1 -> output5/1
  Constant6/1 -> output6/1
  Constant7/1 -> output7/1
  Constant8/1 -> output8/1

== system DDCU_wxt_v02_forA_OpenLoop/OutputSignalProcess/VCU_MCU1_replace/M1SpeedLimit ==
  M1SpeedLimit : Inport
  BitCov : DataTypeConversion  OutDataTypeStr=uint8
  Constant{1..2,5..8} (6 alike) : Constant  Value=0  OutDataTypeStr=uint8
  M1SpeedLimitCOV : DataTypeConversion  OutDataTypeStr=uint8
  M1SpeedLimitRon : Rounding  Operator=round
  M1SpeedLimit_1sat : Saturate  UpperLimit=16380  LowerLimit=0
  M1SpeedLimit_And : simulink/Logic and Bit Operations/Bitwise Operator  logicop=AND  UseBitMask=off  NumInputPorts=2  BitMask=bin2dec('11011001')  BitMaskRealWorld=Stored Integer
  M1SpeedLimit_And_C : Constant  Value=255  OutDataTypeStr=uint32
  M1SpeedLimit_Convert : DataTypeConversion  OutDataTypeStr=uint32
  M1SpeedLimit_D : Product  Inputs=*/
  M1SpeedLimit_D1 : Product  Inputs=*/
  M1SpeedLimit_F : Constant  Value=5  OutDataTypeStr=single
  M1SpeedLimit_L : simulink/Logic and Bit Operations/Bitwise Operator  logicop=AND  UseBitMask=on  BitMask=16380  BitMaskRealWorld=Stored Integer
  M1SpeedLimit_O : Constant  Value=0  OutDataTypeStr=single
  M1SpeedLimit_S : ArithShift  BitShiftNumber=-2
  M1SpeedLimit_sat : Saturate  UpperLimit=20475  LowerLimit=0
  M1SpeedLimit_st : Sum  Inputs=+-
  M1SpeedLimitoutput4_C : Constant  Value=256
  output1 : Outport
  output2 : Outport  Port=2
  output3 : Outport  Port=3
  output4 : Outport  Port=4
  output5 : Outport  Port=5
  output6 : Outport  Port=6
  output7 : Outport  Port=7
  output8 : Outport  Port=8
  wires:
  M1SpeedLimit/1 -> M1SpeedLimit_sat/1
  M1SpeedLimit_sat/1 -> M1SpeedLimit_st/1
  M1SpeedLimit_O/1 -> M1SpeedLimit_st/2
  M1SpeedLimit_st/1 -> M1SpeedLimit_D/1
  M1SpeedLimit_F/1 -> M1SpeedLimit_D/2
  M1SpeedLimit_D/1 -> M1SpeedLimitRon/1
  M1SpeedLimitRon/1 -> M1SpeedLimit_S/1
  M1SpeedLimit_S/1 -> M1SpeedLimit_1sat/1
  M1SpeedLimit_1sat/1 -> M1SpeedLimit_Convert/1
  M1SpeedLimit_Convert/1 -> M1SpeedLimit_L/1
  M1SpeedLimit_L/1 -> M1SpeedLimit_D1/1, M1SpeedLimit_And/1
  M1SpeedLimitoutput4_C/1 -> M1SpeedLimit_D1/2
  M1SpeedLimit_D1/1 -> M1SpeedLimitCOV/1
  M1SpeedLimitCOV/1 -> output4/1
  M1SpeedLimit_And_C/1 -> M1SpeedLimit_And/2
  M1SpeedLimit_And/1 -> BitCov/1
  BitCov/1 -> output3/1
  Constant1/1 -> output1/1
  Constant2/1 -> output2/1
  Constant5/1 -> output5/1
  Constant6/1 -> output6/1
  Constant7/1 -> output7/1
  Constant8/1 -> output8/1

== system DDCU_wxt_v02_forA_OpenLoop/OutputSignalProcess/VCU_MCU1_replace/M1SpeedSet ==
  M1SpeedSet : Inport
  Constant{4..8} (5 alike) : Constant  Value=0  OutDataTypeStr=uint8
  M1SpeedSetBitCov : DataTypeConversion  OutDataTypeStr=uint32
  M1SpeedSetBitCov1 : DataTypeConversion  OutDataTypeStr=uint8
  M1SpeedSetCOV : DataTypeConversion  OutDataTypeStr=uint8
  M1SpeedSetCOV1 : DataTypeConversion  OutDataTypeStr=uint8
  M1SpeedSetRon : Rounding  Operator=round
  M1SpeedSet_1sat : Saturate  UpperLimit=262080  LowerLimit=0
  M1SpeedSet_And : simulink/Logic and Bit Operations/Bitwise Operator  logicop=AND  UseBitMask=off  NumInputPorts=2  BitMask=bin2dec('11011001')  BitMaskRealWorld=Stored Integer
  M1SpeedSet_And1 : simulink/Logic and Bit Operations/Bitwise Operator  logicop=AND  UseBitMask=off  NumInputPorts=2  BitMask=bin2dec('11011001')  BitMaskRealWorld=Stored Integer
  M1SpeedSet_And1_C : Constant  Value=255  OutDataTypeStr=uint32
  M1SpeedSet_And_C : Constant  Value=65535
  M1SpeedSet_Convert : DataTypeConversion  OutDataTypeStr=uint32
  M1SpeedSet_D : Product  Inputs=*/
  M1SpeedSet_D1 : Product  Inputs=*/
  M1SpeedSet_D2 : Product  Inputs=*/
  M1SpeedSet_F : Constant  Value=5  OutDataTypeStr=single
  M1SpeedSet_L : simulink/Logic and Bit Operations/Bitwise Operator  logicop=AND  UseBitMask=on  BitMask=262080  BitMaskRealWorld=Stored Integer
  M1SpeedSet_O : Constant  Value=-5000  OutDataTypeStr=single
  M1SpeedSet_S : ArithShift  BitShiftNumber=-6
  M1SpeedSet_sat : Saturate  UpperLimit=15475  LowerLimit=-5000
  M1SpeedSet_st : Sum  Inputs=+-
  M1SpeedSetoutput2_C : Constant  Value=256
  M1SpeedSetoutput3_C : Constant  Value=65536
  output1 : Outport
  output2 : Outport  Port=2
  output3 : Outport  Port=3
  output4 : Outport  Port=4
  output5 : Outport  Port=5
  output6 : Outport  Port=6
  output7 : Outport  Port=7
  output8 : Outport  Port=8
  wires:
  M1SpeedSet/1 -> M1SpeedSet_sat/1
  M1SpeedSet_sat/1 -> M1SpeedSet_st/1
  M1SpeedSet_O/1 -> M1SpeedSet_st/2
  M1SpeedSet_st/1 -> M1SpeedSet_D/1
  M1SpeedSet_F/1 -> M1SpeedSet_D/2
  M1SpeedSet_D/1 -> M1SpeedSetRon/1
  M1SpeedSetRon/1 -> M1SpeedSet_S/1
  M1SpeedSet_S/1 -> M1SpeedSet_1sat/1
  M1SpeedSet_1sat/1 -> M1SpeedSet_Convert/1
  M1SpeedSet_Convert/1 -> M1SpeedSet_L/1
  M1SpeedSet_L/1 -> M1SpeedSet_D1/1, M1SpeedSet_And/1, M1SpeedSet_And1/1
  M1SpeedSetoutput3_C/1 -> M1SpeedSet_D1/2
  M1SpeedSet_D1/1 -> M1SpeedSetCOV/1
  M1SpeedSetCOV/1 -> output3/1
  M1SpeedSet_And_C/1 -> M1SpeedSetBitCov/1
  M1SpeedSetBitCov/1 -> M1SpeedSet_And/2
  M1SpeedSet_And/1 -> M1SpeedSet_D2/1
  M1SpeedSetoutput2_C/1 -> M1SpeedSet_D2/2
  M1SpeedSet_D2/1 -> M1SpeedSetCOV1/1
  M1SpeedSetCOV1/1 -> output2/1
  M1SpeedSet_And1_C/1 -> M1SpeedSet_And1/2
  M1SpeedSet_And1/1 -> M1SpeedSetBitCov1/1
  M1SpeedSetBitCov1/1 -> output1/1
  Constant4/1 -> output4/1
  Constant5/1 -> output5/1
  Constant6/1 -> output6/1
  Constant7/1 -> output7/1
  Constant8/1 -> output8/1

== system DDCU_wxt_v02_forA_OpenLoop/OutputSignalProcess/VCU_MCU1_replace/M2Drive ==
  M2Drive : Inport
  Constant{1..4,6..8} (7 alike) : Constant  Value=0  OutDataTypeStr=uint8
  M2DriveRon : Rounding  Operator=round
  M2Drive_1sat : Saturate  UpperLimit=12  LowerLimit=0
  M2Drive_Convert : DataTypeConversion  OutDataTypeStr=uint8
  M2Drive_Convert1 : DataTypeConversion  OutDataTypeStr=uint32
  M2Drive_D : Product  Inputs=*/
  M2Drive_F : Constant  OutDataTypeStr=single
  M2Drive_L : simulink/Logic and Bit Operations/Bitwise Operator  logicop=AND  UseBitMask=on  BitMask=12  BitMaskRealWorld=Stored Integer
  M2Drive_O : Constant  Value=0  OutDataTypeStr=single
  M2Drive_S : ArithShift  BitShiftNumber=-2
  M2Drive_sat : Saturate  UpperLimit=3  LowerLimit=0
  M2Drive_st : Sum  Inputs=+-
  output1 : Outport
  output2 : Outport  Port=2
  output3 : Outport  Port=3
  output4 : Outport  Port=4
  output5 : Outport  Port=5
  output6 : Outport  Port=6
  output7 : Outport  Port=7
  output8 : Outport  Port=8
  wires:
  M2Drive/1 -> M2Drive_sat/1
  M2Drive_sat/1 -> M2Drive_st/1
  M2Drive_O/1 -> M2Drive_st/2
  M2Drive_st/1 -> M2Drive_D/1
  M2Drive_F/1 -> M2Drive_D/2
  M2Drive_D/1 -> M2DriveRon/1
  M2DriveRon/1 -> M2Drive_S/1
  M2Drive_S/1 -> M2Drive_1sat/1
  M2Drive_1sat/1 -> M2Drive_Convert1/1
  M2Drive_Convert1/1 -> M2Drive_L/1
  M2Drive_L/1 -> M2Drive_Convert/1
  M2Drive_Convert/1 -> output5/1
  Constant1/1 -> output1/1
  Constant2/1 -> output2/1
  Constant3/1 -> output3/1
  Constant4/1 -> output4/1
  Constant6/1 -> output6/1
  Constant7/1 -> output7/1
  Constant8/1 -> output8/1

== system DDCU_wxt_v02_forA_OpenLoop/OutputSignalProcess/VCU_MCU1_replace/M2Enable ==
  M2Enable : Inport
  Constant{1..3,5..8} (7 alike) : Constant  Value=0  OutDataTypeStr=uint8
  M2EnableRon : Rounding  Operator=round
  M2Enable_1sat : Saturate  UpperLimit=192  LowerLimit=0
  M2Enable_Convert : DataTypeConversion  OutDataTypeStr=uint8
  M2Enable_Convert1 : DataTypeConversion  OutDataTypeStr=uint32
  M2Enable_D : Product  Inputs=*/
  M2Enable_F : Constant  OutDataTypeStr=single
  M2Enable_L : simulink/Logic and Bit Operations/Bitwise Operator  logicop=AND  UseBitMask=on  BitMask=192  BitMaskRealWorld=Stored Integer
  M2Enable_O : Constant  Value=0  OutDataTypeStr=single
  M2Enable_S : ArithShift  BitShiftNumber=-6
  M2Enable_sat : Saturate  UpperLimit=3  LowerLimit=0
  M2Enable_st : Sum  Inputs=+-
  output1 : Outport
  output2 : Outport  Port=2
  output3 : Outport  Port=3
  output4 : Outport  Port=4
  output5 : Outport  Port=5
  output6 : Outport  Port=6
  output7 : Outport  Port=7
  output8 : Outport  Port=8
  wires:
  M2Enable/1 -> M2Enable_sat/1
  M2Enable_sat/1 -> M2Enable_st/1
  M2Enable_O/1 -> M2Enable_st/2
  M2Enable_st/1 -> M2Enable_D/1
  M2Enable_F/1 -> M2Enable_D/2
  M2Enable_D/1 -> M2EnableRon/1
  M2EnableRon/1 -> M2Enable_S/1
  M2Enable_S/1 -> M2Enable_1sat/1
  M2Enable_1sat/1 -> M2Enable_Convert1/1
  M2Enable_Convert1/1 -> M2Enable_L/1
  M2Enable_L/1 -> M2Enable_Convert/1
  M2Enable_Convert/1 -> output4/1
  Constant1/1 -> output1/1
  Constant2/1 -> output2/1
  Constant3/1 -> output3/1
  Constant5/1 -> output5/1
  Constant6/1 -> output6/1
  Constant7/1 -> output7/1
  Constant8/1 -> output8/1
